simulink model "modulo"  (R2020a)
settings: Solver=VariableStepAuto  StartTime=0.0  StopTime=0.01  RelTol=1e-3
values from neighbouring files (symbols this model uses):
  ts_send = 0.01    [main.m]
libraries: powerlib_meascontrol x9, powerlib x6, instrumentlib x2, simulink x1
settings Model: Creator=bazur  LastModifiedBy=bazur

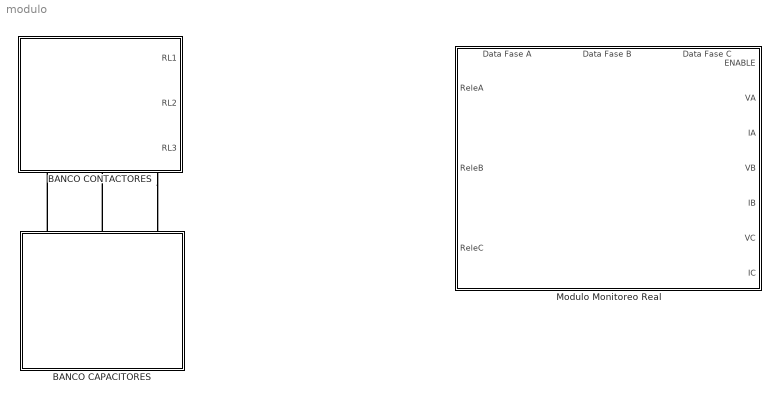
== system modulo ==
  BANCO CAPACITORES : Subsystem
      mask Display: image('C:\Users\bazur\Desktop\RedNeuronal\RedNeuronalTesis\matlab\pictures\capacitores.jpg'); % Use "Edit Image" on toolstrip to change.
  BANCO CONTACTORES : Subsystem
      settings: PortSchema="{\"entries\":[{\"content\":{\"sides\":[{\"content\":{\"connectorIds\":[\"LConn1\",\"LConn2\",\"LConn3\"]},\"type\":\"ConnectorPlacement.EquallySpacedRectSide\",\"uuid\":\"e80dd9a9-4bfc-4eab-a7c4-3db18c523d34\"},{\"content\":{\"connectorIds\":[\"RConn1\",\"RConn2\",\"RConn3\"],\"side\":\"RIGHT\"},\"type\":\"ConnectorPlacement.EquallySpacedRectSide\",\"uuid\":\"979478e7-303b-4584-8727-188264d935b7\"},{\"content\":{\"connectorIds\":[],\"side\":\"TOP\"},\"type\":\"ConnectorPlacement.EquallySpacedRectSide\",\"uuid\":\"a9ebe4a2-f61b-43c6-b574-20dbaa59ac96\"},{\"content\":{\"connectorIds\":[\"In1\",\"In2\",\"In3\"],\"side\":\"BOTTOM\"},\"type\":\"ConnectorPlacement.EquallySpacedRectSide\",\"uuid\":\"4a287abd-7c31-4709-8be9-666923cac126\"}]},\"type\":\"ConnectorPlacement.EquallySpacedConnector\",\"uuid\":\"5e3ed12c-fb1f-449d-870e-ded7ccdc4ac0\"}],\"packageUris\":[\"http://schema.mathworks.com/mf0/Connector/19700101\"],\"version\":\"1.0\"}"
      mask Display: image('C:\Users\bazur\Desktop\RedNeuronal\RedNeuronalTesis\matlab\pictures\contactores.png'); % Use "Edit Image" on toolstrip to change.
  Modulo Monitoreo Real : Subsystem
      settings: PortSchema="{\"entries\":[{\"content\":{\"sides\":[{\"content\":{\"connectorIds\":[\"In1\",\"In2\",\"In3\",\"In4\",\"In5\",\"In6\",\"In7\"]},\"type\":\"ConnectorPlacement.EquallySpacedRectSide\",\"uuid\":\"f726b031-035b-4703-af3f-a4e51d0dca98\"},{\"content\":{\"connectorIds\":[\"Out1\",\"Out2\",\"Out3\"],\"side\":\"RIGHT\"},\"type\":\"ConnectorPlacement.EquallySpacedRectSide\",\"uuid\":\"d317a734-42d7-4878-a87e-3ae99e4df09f\"},{\"content\":{\"connectorIds\":[\"Out4\",\"Out5\",\"Out6\"],\"side\":\"TOP\"},\"type\":\"ConnectorPlacement.EquallySpacedRectSide\",\"uuid\":\"3f8ce4c0-84cc-4512-a908-abb1f3fc3c08\"},{\"content\":{\"connectorIds\":[],\"side\":\"BOTTOM\"},\"type\":\"ConnectorPlacement.EquallySpacedRectSide\",\"uuid\":\"95f59266-31ff-4071-9e63-6fbc8f4be1bf\"}]},\"type\":\"ConnectorPlacement.EquallySpacedConnector\",\"uuid\":\"51425b5b-918b-4ee3-8f8a-3aaf36556f32\"}],\"packageUris\":[\"http://schema.mathworks.com/mf0/Connector/19700101\"],\"version\":\"1.0\"}"
      mask Display: image('C:\Users\bazur\Desktop\RedNeuronal\RedNeuronalTesis\matlab\pictures\modulo.jpg'); % Use "Edit Image" on toolstrip to change.
  connections:
  BANCO CAPACITORES/LConn1 -- BANCO CONTACTORES/RConn1
  BANCO CAPACITORES/LConn2 -- BANCO CONTACTORES/RConn2
  BANCO CONTACTORES/RConn3 -- BANCO CAPACITORES/LConn3

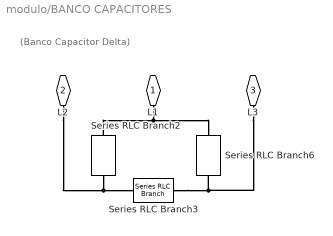
== system modulo/BANCO CAPACITORES ==
  note: (Banco Capacitor Delta)
  Series RLC Branch2 : powerlib/Elements/Series RLC Branch  LConnTagsString=__new0  RConnTagsString=__new0  BranchType=C  Resistance=1  Inductance=1e-3  SetiL0=off  InitialCurrent=0  Capacitance=0.006  Setx0=off  InitialVoltage=0  Measurements=None
  Series RLC Branch3 : powerlib/Elements/Series RLC Branch  LConnTagsString=__new0  RConnTagsString=__new0  BranchType=C  Resistance=1  Inductance=1e-3  SetiL0=off  InitialCurrent=0  Capacitance=0.006  Setx0=off  InitialVoltage=0  Measurements=None
  Series RLC Branch6 : powerlib/Elements/Series RLC Branch  LConnTagsString=__new0  RConnTagsString=__new0  BranchType=C  Resistance=1  Inductance=1e-3  SetiL0=off  InitialCurrent=0  Capacitance=0.006  Setx0=off  InitialVoltage=0  Measurements=None
  L1 : PMIOPort  Side=Left
  L2 : PMIOPort  Port=2  Side=Left
  L3 : PMIOPort  Port=3  Side=Left
  connections:
  Series RLC Branch2/LConn1 -- Series RLC Branch6/LConn1 -- L1/RConn1
  Series RLC Branch2/RConn1 -- L2/RConn1 -- Series RLC Branch3/LConn1
  Series RLC Branch3/RConn1 -- L3/RConn1 -- Series RLC Branch6/RConn1

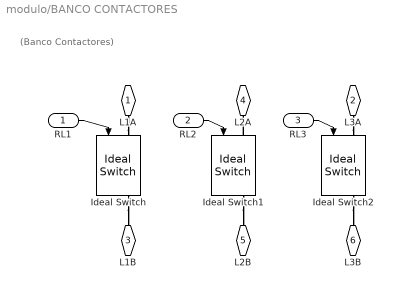
== system modulo/BANCO CONTACTORES ==
  note: (Banco Contactores)
  RL1 : Inport
  RL2 : Inport  Port=2
  RL3 : Inport  Port=3
  Ideal Switch : powerlib/Power Electronics/Ideal Switch  Ron=0.001  Lon=0  IC=0  Rs=1e5  Cs=inf  Measurements=on
  Ideal Switch1 : powerlib/Power Electronics/Ideal Switch  Ron=0.001  Lon=0  IC=0  Rs=1e5  Cs=inf  Measurements=on
  Ideal Switch2 : powerlib/Power Electronics/Ideal Switch  Ron=0.001  Lon=0  IC=0  Rs=1e5  Cs=inf  Measurements=on
  L1A : PMIOPort  Side=Left
  L3A : PMIOPort  Port=2  Side=Left
  L1B : PMIOPort  Port=3  Side=Left
  L2A : PMIOPort  Port=4  Side=Right
  L2B : PMIOPort  Port=5  Side=Right
  L3B : PMIOPort  Port=6  Side=Right
  wires:
  RL1/1 -> Ideal Switch/1
  RL2/1 -> Ideal Switch1/1
  RL3/1 -> Ideal Switch2/1
  connections:
  L1A/RConn1 -- Ideal Switch/LConn1
  Ideal Switch1/LConn1 -- L2A/RConn1
  L3A/RConn1 -- Ideal Switch2/LConn1
  Ideal Switch/RConn1 -- L1B/RConn1
  Ideal Switch1/RConn1 -- L2B/RConn1
  Ideal Switch2/RConn1 -- L3B/RConn1

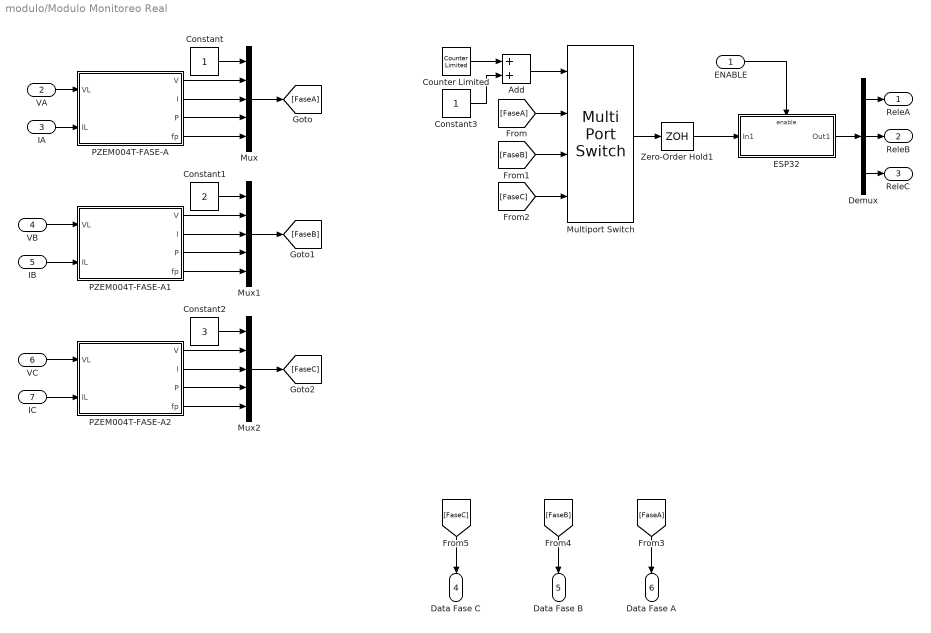
== system modulo/Modulo Monitoreo Real ==
  ENABLE : Inport
  VA : Inport  Port=2
  IA : Inport  Port=3
  VB : Inport  Port=4
  IB : Inport  Port=5
  VC : Inport  Port=6
  IC : Inport  Port=7
  Add : Sum
  Constant : Constant
  Constant1 : Constant  Value=2
  Constant2 : Constant  Value=3
  Constant3 : Constant
  Counter Limited : simulink/Sources/Counter Limited  uplimit=2  tsamp=ts_send
  Demux : Demux  Outputs=3
  ESP32 : Subsystem  TreatAsAtomicUnit=on
  Multiport Switch : MultiPortSwitch
  Mux : Mux  Inputs=5
  Mux1 : Mux  Inputs=5
  Mux2 : Mux  Inputs=5
  PZEM004T-FASE-A : Subsystem
      mask Display: image('C:\Users\bazur\Desktop\RedNeuronal\RedNeuronalTesis\matlab\pictures\PZEM-004-module.jpg'); % Use "Edit Image" on toolstrip to change.
  PZEM004T-FASE-A1 : Subsystem
      mask Display: image('C:\Users\bazur\Desktop\RedNeuronal\RedNeuronalTesis\matlab\pictures\PZEM-004-module.jpg'); % Use "Edit Image" on toolstrip to change.
  PZEM004T-FASE-A2 : Subsystem
      mask Display: image('C:\Users\bazur\Desktop\RedNeuronal\RedNeuronalTesis\matlab\pictures\PZEM-004-module.jpg'); % Use "Edit Image" on toolstrip to change.
  Zero-Order Hold1 : ZeroOrderHold  SampleTime=ts_send
  ReleA : Outport
  ReleB : Outport  Port=2
  ReleC : Outport  Port=3
  Data Fase C : Outport  Port=4
  Data Fase B : Outport  Port=5
  Data Fase A : Outport  Port=6
  wires:
  VA/1 -> PZEM004T-FASE-A/1(VL)
  IA/1 -> PZEM004T-FASE-A/2(IL)
  IB/1 -> PZEM004T-FASE-A1/2(IL)
  VB/1 -> PZEM004T-FASE-A1/1(VL)
  PZEM004T-FASE-A/1(V) -> Mux/2
  PZEM004T-FASE-A/2(I) -> Mux/3
  PZEM004T-FASE-A/3(P) -> Mux/4
  PZEM004T-FASE-A/4(fp) -> Mux/5
  Constant/1 -> Mux/1
  Mux/1 -> [FaseA]
  [FaseA] -> Multiport Switch/2
  Constant1/1 -> Mux1/1
  Mux1/1 -> [FaseB]
  PZEM004T-FASE-A1/2(I) -> Mux1/3
  PZEM004T-FASE-A1/4(fp) -> Mux1/5
  PZEM004T-FASE-A1/1(V) -> Mux1/2
  PZEM004T-FASE-A1/3(P) -> Mux1/4
  Constant2/1 -> Mux2/1
  VC/1 -> PZEM004T-FASE-A2/1(VL)
  PZEM004T-FASE-A2/3(P) -> Mux2/4
  IC/1 -> PZEM004T-FASE-A2/2(IL)
  PZEM004T-FASE-A2/4(fp) -> Mux2/5
  PZEM004T-FASE-A2/1(V) -> Mux2/2
  Mux2/1 -> [FaseC]
  PZEM004T-FASE-A2/2(I) -> Mux2/3
  [FaseB] -> Multiport Switch/3
  [FaseC] -> Multiport Switch/4
  Counter Limited/1 -> Add/1
  Add/1 -> Multiport Switch/1
  Constant3/1 -> Add/2
  Multiport Switch/1 -> Zero-Order Hold1/1
  [FaseB] -> Data Fase B/1
  [FaseC] -> Data Fase C/1
  Demux/2 -> ReleB/1
  Demux/1 -> ReleA/1
  Demux/3 -> ReleC/1
  [FaseA] -> Data Fase A/1
  Zero-Order Hold1/1 -> ESP32/1(In1)
  ESP32/1(Out1) -> Demux/1
  ENABLE/1 -> ESP32/Enable

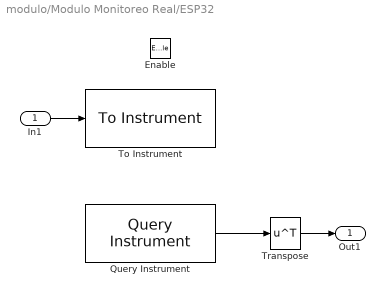
== system modulo/Modulo Monitoreo Real/ESP32 ==
  In1 : Inport
  Enable : EnablePort
  Query Instrument : instrumentlib/Query Instrument  sampleTime=ts_read  isWorkspaceObject=off  timeout=10  inputBufferSize=1012  protocol=Serial  serialPort=COM1  baudRate=115200  gpibVendor=Keysight Technologies  boardIndex=0  primaryAddress=1  secondaryAddress=0  visaVendor=Keysight  visaSerialPort=0  chassisIndex=0  logicalAddress=0  tcpRemoteHost='127.0.0.1'  tcpRemotePort=4500  udpRemoteHost='127.0.0.1'  udpRemotePort=9090  visaTCPBoardIndex=0  visaTCPRemoteHost='127.0.0.1'  usbBoardIndex=0  usbManufID=0  usbModelCode=0  usbSerialNumber=0  initAction=None  initCommand='DATA:SOURCE CH1'  initFunction=get  queryCommand='rele\n'  responseFormat=ASCII  asciiFormatting=ASCII_read  precision=8-bit integer  byteOrder=Little endian  valuesToRead=1  removeBytes=off  afterOutputAction=Repeat query for new data  enableFrames=on  frameSize=3
      settings: SourceProductBaseCode=IC
  To Instrument : instrumentlib/To Instrument  sampleTime=ts_send  isWorkspaceObject=off  timeout=10  inputBufferSize=725000  protocol=Serial  serialPort=COM1  baudRate=115200  gpibVendor=ICS Electronics  boardIndex=0  primaryAddress=1  secondaryAddress=0  visaVendor=Keysight  visaSerialPort=0  chassisIndex=0  logicalAddress=0  tcpRemoteHost='127.0.0.1'  tcpRemotePort=4500  udpRemoteHost='127.0.0.1'  udpRemotePort=9090  visaTCPBoardIndex=0  visaTCPRemoteHost='127.0.0.1'  usbBoardIndex=0  usbManufID=0  usbModelCode=0  usbSerialNumber=0  initAction=None  initCommand='DATA:SOURCE CH1'  initFunction=get  command=''  sendFormat=ASCII  asciiFormatting=ASCII_send  precision=8-bit integer  byteOrder=Little endian
      settings: SourceProductBaseCode=IC
  Transpose : Math  Operator=transpose  SaturateOnIntegerOverflow=on
  Out1 : Outport
  wires:
  Query Instrument/1 -> Transpose/1
  In1/1 -> To Instrument/1
  Transpose/1 -> Out1/1

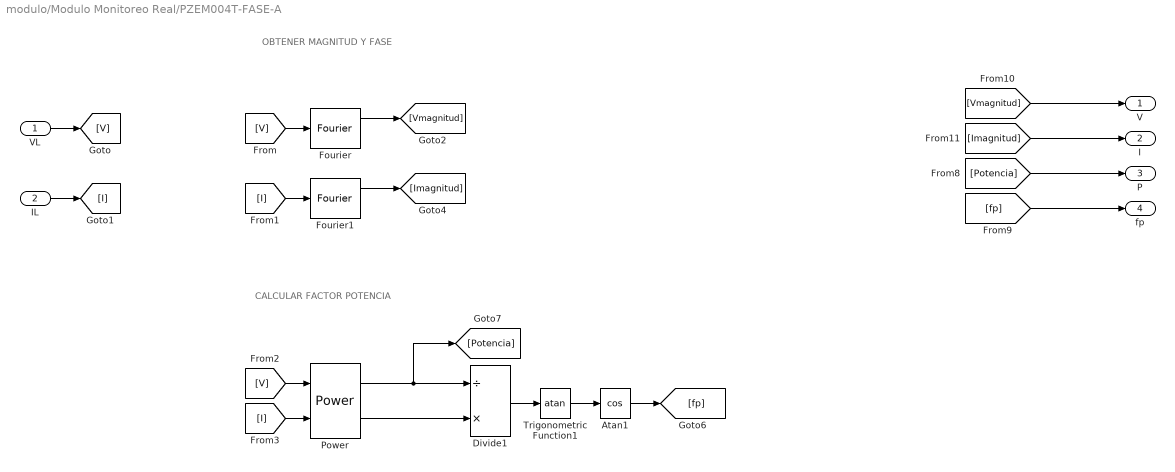
== system modulo/Modulo Monitoreo Real/PZEM004T-FASE-A ==
  note: OBTENER MAGNITUD Y FASE
  note: CALCULAR FACTOR POTENCIA
  VL : Inport
  IL : Inport  Port=2
  Atan1 : Trigonometry  Operator=cos
  Divide1 : Product  Inputs=/*
  Fourier : powerlib_meascontrol/Measurements/Fourier  Freq=60  n=1  InInit=[0, 0]  Ts=0
  Fourier1 : powerlib_meascontrol/Measurements/Fourier  Freq=60  n=1  InInit=[0, 0]  Ts=0
  Power : powerlib_meascontrol/Measurements/Power  Freq=60  Vinit=[1, 0]  Iinit=[1, 0]  Ts=0
  Trigonometric Function1 : Trigonometry  Operator=atan
  V : Outport
  I : Outport  Port=2
  P : Outport  Port=3
  fp : Outport  Port=4
  wires:
  VL/1 -> [V]
  [V] -> Fourier/1
  IL/1 -> [I]
  [I] -> Fourier1/1
  Fourier/1 -> [Vmagnitud]
  Fourier1/1 -> [Imagnitud]
  [Vmagnitud] -> V/1
  [Imagnitud] -> I/1
  [fp] -> fp/1
  [Potencia] -> P/1
  Divide1/1 -> Trigonometric Function1/1
  Power/2 -> Divide1/2
  Power/1 -> [Potencia], Divide1/1
  Trigonometric Function1/1 -> Atan1/1
  [V] -> Power/1
  [I] -> Power/2
  Atan1/1 -> [fp]

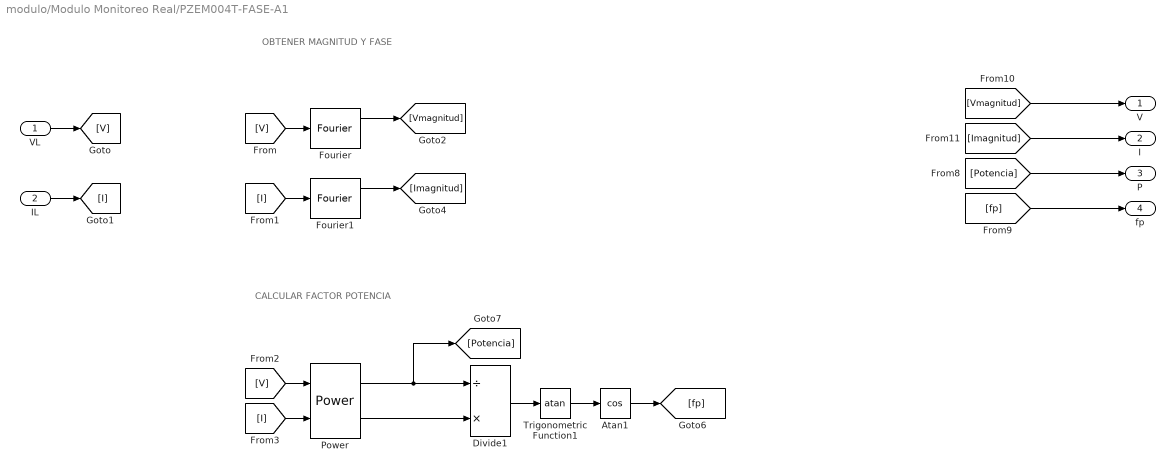
== system modulo/Modulo Monitoreo Real/PZEM004T-FASE-A1 ==
  note: OBTENER MAGNITUD Y FASE
  note: CALCULAR FACTOR POTENCIA
  VL : Inport
  IL : Inport  Port=2
  Atan1 : Trigonometry  Operator=cos
  Divide1 : Product  Inputs=/*
  Fourier : powerlib_meascontrol/Measurements/Fourier  Freq=60  n=1  InInit=[0, 0]  Ts=0
  Fourier1 : powerlib_meascontrol/Measurements/Fourier  Freq=60  n=1  InInit=[0, 0]  Ts=0
  Power : powerlib_meascontrol/Measurements/Power  Freq=60  Vinit=[1, 0]  Iinit=[1, 0]  Ts=0
  Trigonometric Function1 : Trigonometry  Operator=atan
  V : Outport
  I : Outport  Port=2
  P : Outport  Port=3
  fp : Outport  Port=4
  wires:
  VL/1 -> [V]
  [V] -> Fourier/1
  IL/1 -> [I]
  [I] -> Fourier1/1
  Fourier/1 -> [Vmagnitud]
  Fourier1/1 -> [Imagnitud]
  [Vmagnitud] -> V/1
  [Imagnitud] -> I/1
  [fp] -> fp/1
  [Potencia] -> P/1
  Divide1/1 -> Trigonometric Function1/1
  Power/2 -> Divide1/2
  Power/1 -> [Potencia], Divide1/1
  Trigonometric Function1/1 -> Atan1/1
  [V] -> Power/1
  [I] -> Power/2
  Atan1/1 -> [fp]

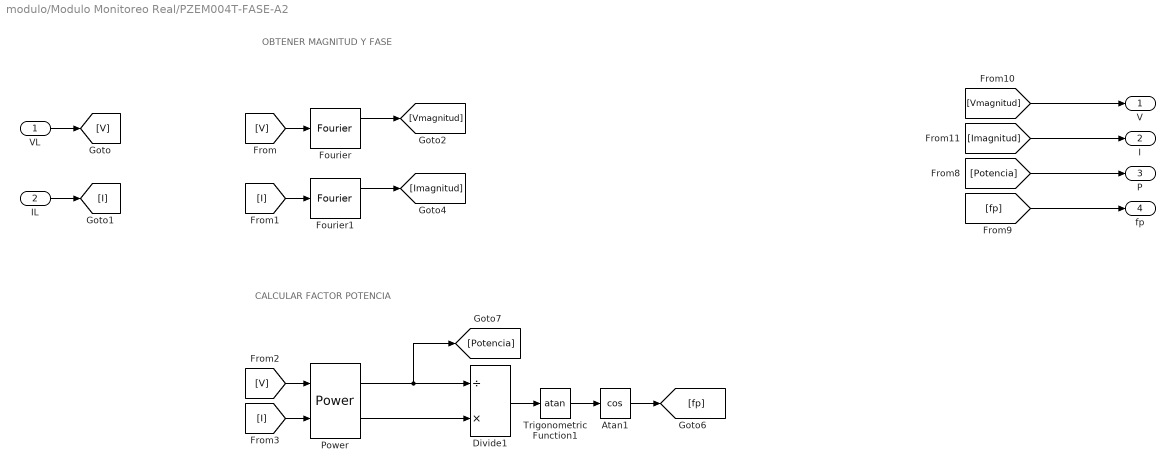
== system modulo/Modulo Monitoreo Real/PZEM004T-FASE-A2 ==
  note: OBTENER MAGNITUD Y FASE
  note: CALCULAR FACTOR POTENCIA
  VL : Inport
  IL : Inport  Port=2
  Atan1 : Trigonometry  Operator=cos
  Divide1 : Product  Inputs=/*
  Fourier : powerlib_meascontrol/Measurements/Fourier  Freq=60  n=1  InInit=[0, 0]  Ts=0
  Fourier1 : powerlib_meascontrol/Measurements/Fourier  Freq=60  n=1  InInit=[0, 0]  Ts=0
  Power : powerlib_meascontrol/Measurements/Power  Freq=60  Vinit=[1, 0]  Iinit=[1, 0]  Ts=0
  Trigonometric Function1 : Trigonometry  Operator=atan
  V : Outport
  I : Outport  Port=2
  P : Outport  Port=3
  fp : Outport  Port=4
  wires:
  VL/1 -> [V]
  [V] -> Fourier/1
  IL/1 -> [I]
  [I] -> Fourier1/1
  Fourier/1 -> [Vmagnitud]
  Fourier1/1 -> [Imagnitud]
  [Vmagnitud] -> V/1
  [Imagnitud] -> I/1
  [fp] -> fp/1
  [Potencia] -> P/1
  Divide1/1 -> Trigonometric Function1/1
  Power/2 -> Divide1/2
  Power/1 -> [Potencia], Divide1/1
  Trigonometric Function1/1 -> Atan1/1
  [V] -> Power/1
  [I] -> Power/2
  Atan1/1 -> [fp]
